simulink model "water_hopper_fix"  (Simulink 7.9)
settings: Solver=ode23t  StartTime=0.0  StopTime=5  MaxStep=1e-3  RelTol=1e-3
values from neighbouring files (symbols this model uses):
  Amp = AMP(jj,1)    [TwoD_search.m]
  C_d = 0.703    [SimParam.m]
  density = 1000    [SimParam.m]
  freq = FREQ(1,kk)    [TwoD_search.m]
  g = 9.81    [SimParam.m]
  h0 = leg_length    [TwoD_search.m]
  leg_length = 0.06    [SimParam.m]
  mass = 0.05    [SimParam.m]
  S1 = pi*r1^2    (= 0.00125663706144)    [SimParam.m]
  S2 = pi*r2^2    (= 7.85398163397e-05)    [SimParam.m]
libraries: mblibv1 x13, simulink x1
settings Model: Creator=Metti  LastModifiedBy=Metti
settings SolverCC: ZeroCrossControl=DisableAll
settings ConfigurationSet: Description=SimMechanics 2G

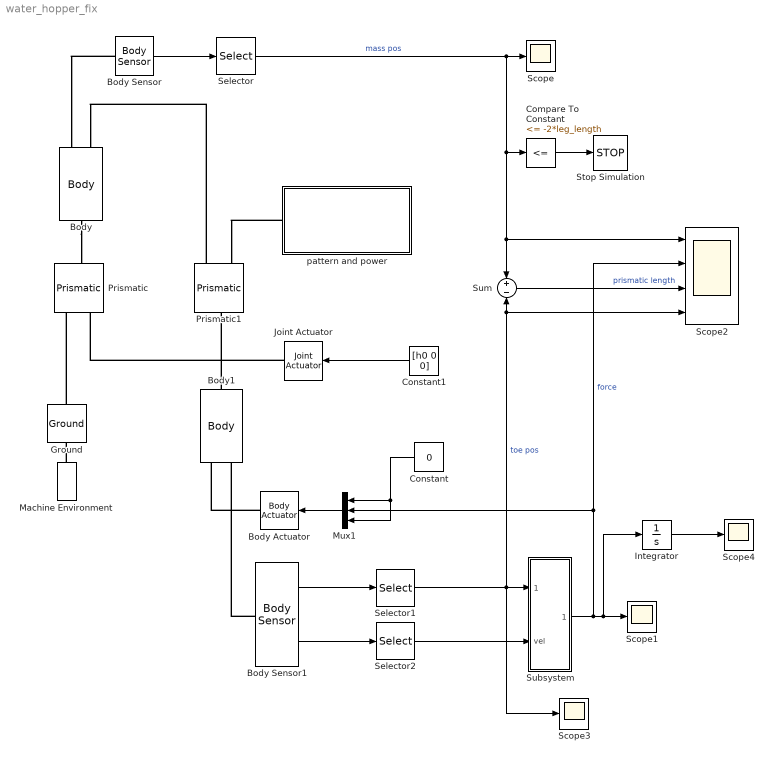
== system water_hopper_fix ==
  Body : mblibv1/Bodies/Body  LConnTagsString=CS1  RConnTagsString=CS2|CS3  UpdateFromCAD=off  DialogClass=MechanicalBodyBlock  Mass=mass  MassUnits=kg  InertiaUnits=kg*m^2  Inertia=eye(3)  Shape=Cylinder  ShapeDims=[1 1]  ShapeUnits=m  ShapeUse=false  Density=1  DensityUnits=kg/m^3  DensityUse=false  GraphicsMode=MACHINE_DEFAULT  BodyColorSelMode=MACHINE_DEFAULT  BodyColor=[1 0 0]  AttachedToCS=CG  CG=Left$CG$[0 0 0]$WORLD$WORLD$m$[0 0 0]$Euler X-Y-Z$deg$WORLD$false$none  WorkingFrames=Left$CS1$[0 0 0]$CG$CG$m$[0 0 0]$Euler X-Y-Z$deg$WORLD$true$none#Right$CS2$[0 0 0]$CG$CG$m$[0 0 0]$Euler X-Y-Z$deg$WORLD$true$none#Right$CS3$[0 0 0]$CG$CG$m$[0 0 0]$Euler X-Y-Z$deg$WORLD$true$none  CGPos=[0 0 0]  CGRot=[0 0 0]  CS0Pos=[]  CS0Rot=[]  CS1Pos=[0 0 0]  CS1Rot=[0 0 0]  CS2Pos=[0 0 0]  CS2Rot=[0 0 0]  CS3Pos=[0 0 0]  CS3Rot=[0 0 0]  CS4Pos=[]  CS4Rot=[]  CS5Pos=[]  CS5Rot=[]  CS6Pos=[]  CS6Rot=[]  CS7Pos=[]  CS7Rot=[]  CS8Pos=[]  CS8Rot=[]  CS9Pos=[]  CS9Rot=[]  CS10Pos=[]  CS10Rot=[]  CS11Pos=[]  CS11Rot=[]  CS12Pos=[]  CS12Rot=[]  CS13Pos=[]  CS13Rot=[]  CS14Pos=[]  CS14Rot=[]  CS15Pos=[]  CS15Rot=[]  CS16Pos=[]  CS16Rot=[]  CS17Pos=[]  CS17Rot=[]  CS18Pos=[]  CS18Rot=[]  CS19Pos=[]  CS19Rot=[]  CS20Pos=[]  CS20Rot=[]
  Body Actuator : mblibv1/Sensors &  Actuators/Body Actuator  UpdateFromCAD=off  PhysicalDomain=Mechanical  PortType=blob  ActuationStyle=Force  AngleUnits=deg  ArcVelocityUnits=deg/s  ArcAccelerationUnits=deg/s^2  CoordPositionUnits=m  VelocityUnits=m/s  AccelerationUnits=m/s^2  ForceUnits=N  TorqueUnits=N-m  ActiveIO=on  Width=3  DialogClass=MechanicalActuatorBlock  ReferenceFrame=Absolute (World)  Angle=off  CoordPosition=on  Force=on  Torque=off
  Body Sensor : mblibv1/Sensors &  Actuators/Body Sensor  UpdateFromCAD=off  PhysicalDomain=Mechanical  PortType=blob  Muxed=on  Pose=off  Angle=on  AngleUnits=deg  ArcVelocity=off  ArcVelocityUnits=deg/s  ArcAcceleration=off  ArcAccelerationUnits=deg/s^2  CoordPosition=on  CoordPositionUnits=m  Velocity=off  VelocityUnits=m/s  Acceleration=off  AccelerationUnits=m/s^2  Quaternion=on  QuaternionDT=off  QuaternionDDT=off  QuaternionUnits=off  OutputVector=[1]  ActiveIO=on  Width=3  DialogClass=MechanicalSensorBlock  ReferenceFrame=Absolute (World)
  Body Sensor1 : mblibv1/Sensors &  Actuators/Body Sensor  UpdateFromCAD=off  PhysicalDomain=Mechanical  PortType=blob  Muxed=off  Pose=off  Angle=on  AngleUnits=deg  ArcVelocity=off  ArcVelocityUnits=deg/s  ArcAcceleration=off  ArcAccelerationUnits=deg/s^2  CoordPosition=on  CoordPositionUnits=m  Velocity=on  VelocityUnits=m/s  Acceleration=off  AccelerationUnits=m/s^2  Quaternion=on  QuaternionDT=off  QuaternionDDT=off  QuaternionUnits=off  OutputVector=[1]  ActiveIO=on  Width=6  DialogClass=MechanicalSensorBlock  ReferenceFrame=Absolute (World)
  Body1 : mblibv1/Bodies/Body  LConnTagsString=CS1  RConnTagsString=CS2|CS3  UpdateFromCAD=off  DialogClass=MechanicalBodyBlock  Mass=0  MassUnits=kg  InertiaUnits=kg*m^2  Inertia=eye(3)  Shape=Cylinder  ShapeDims=[1 1]  ShapeUnits=m  ShapeUse=false  Density=1  DensityUnits=kg/m^3  DensityUse=false  GraphicsMode=MACHINE_DEFAULT  BodyColorSelMode=MACHINE_DEFAULT  BodyColor=[1 0 0]  AttachedToCS=CG  CG=Left$CG$[0 -leg_length 0]$CS1$CS1$m$[0 0 0]$Euler X-Y-Z$deg$WORLD$false$none  WorkingFrames=Left$CS1$[0 0 0]$Adjoining$Adjoining$m$[0 0 0]$Euler X-Y-Z$deg$WORLD$true$none#Right$CS2$[0 -leg_length 0]$CS1$CS1$m$[0 0 0]$Euler X-Y-Z$deg$WORLD$true$none#Right$CS3$[0 -leg_length 0]$CS1$CS1$m$[0 0 0]$Euler X-Y-Z$deg$WORLD$true$none  CGPos=[0 -leg_length 0]  CGRot=[0 0 0]  CS0Pos=[]  CS0Rot=[]  CS1Pos=[0 0 0]  CS1Rot=[0 0 0]  CS2Pos=[0 -leg_length 0]  CS2Rot=[0 0 0]  CS3Pos=[0 -leg_length 0]  CS3Rot=[0 0 0]  CS4Pos=[]  CS4Rot=[]  CS5Pos=[]  CS5Rot=[]  CS6Pos=[]  CS6Rot=[]  CS7Pos=[]  CS7Rot=[]  CS8Pos=[]  CS8Rot=[]  CS9Pos=[]  CS9Rot=[]  CS10Pos=[]  CS10Rot=[]  CS11Pos=[]  CS11Rot=[]  CS12Pos=[]  CS12Rot=[]  CS13Pos=[]  CS13Rot=[]  CS14Pos=[]  CS14Rot=[]  CS15Pos=[]  CS15Rot=[]  CS16Pos=[]  CS16Rot=[]  CS17Pos=[]  CS17Rot=[]  CS18Pos=[]  CS18Rot=[]  CS19Pos=[]  CS19Rot=[]  CS20Pos=[]  CS20Rot=[]
  Compare To Constant : simulink/Logic and Bit Operations/Compare To Constant  relop=<=  const=-2*leg_length  OutDataTypeStr=boolean
  Constant : Constant  Value=0
  Constant1 : Constant  Value=[h0 0 0]
  Ground : mblibv1/Bodies/Ground  UpdateFromCAD=off  LeftPortType=env  RightPortType=workingframe  PhysicalDomain=Mechanical  DialogClass=GroundBlock  CoordPosition=[0 0 0]  CoordPositionUnits=m  StateVectorMgrId=3  MachineId=[3 0]  ShowEnvPort=on
  Integrator : Integrator
  Joint Actuator : mblibv1/Sensors &  Actuators/Joint Actuator  UpdateFromCAD=off  PhysicalDomain=Mechanical  PortType=blob  ActuationStyle=Motion  AngleUnits=deg  ArcVelocityUnits=deg/s  ArcAccelerationUnits=deg/s^2  CoordPositionUnits=m  VelocityUnits=m/s  AccelerationUnits=m/s^2  ForceUnits=N  TorqueUnits=N*m  ActiveIO=on  Width=3  DialogClass=MechanicalActuatorBlock  Primitive=P1  ReferenceFrame=Absolute (World)
  Machine Environment : mblibv1/Bodies/Machine Environment  PortType=env  PhysicalDomain=Mechanical  DialogTemplateClass=MECH.MachineEnvironment  SyncWhenCopied=off  Gravity=[0 -g 0]  GravityUnits=m/s^2  GravityAsSignal=off  Dimensionality=Auto-detect  AnalysisType=Forward dynamics  LinearAssemblyTolerance=1e-3  LinearAssemblyToleranceUnits=m  AngularAssemblyTolerance=1e-3  AngularAssemblyToleranceUnits=rad  ConstraintSolverType=Stabilizing  ConstraintRelTolerance=1e-4  ConstraintAbsTolerance=1e-4  UseRobustSingularityHandling=off  RedundancyAnalysisToleranceType=Automatically select tolerance  RedundancyAnalysisTolerance=1e-14  StatePerturbationType=Fixed  PerturbationSize=1e-5  VisualizeMachine=on  BodyVisualizationType=Use model default body geometries  BodyColorSelMode=Use model default  DefaultBodyColor=[1 0 0]
  Mux1 : Mux  Inputs=3
  Prismatic : mblibv1/Joints/Prismatic  LConnTagsString=__newl0|SA1  RConnTagsString=__newr0  UpdateFromCAD=off  NumSAPorts=1  CutJoint=off  MarkAsCut=off  Primitives=prismatic  PrimitiveProps=P1$World$[0 1 0]$prismatic  DialogClass=JointBlock  P1Axis=[0 1 0]
  Prismatic1 : mblibv1/Joints/Prismatic  LConnTagsString=__newl0|SA1  RConnTagsString=__newr0  UpdateFromCAD=off  NumSAPorts=1  CutJoint=off  MarkAsCut=off  Primitives=prismatic  PrimitiveProps=P1$World$[0 1 0]$prismatic  DialogClass=JointBlock  P1Axis=[0 1 0]
  Scope{,1,3..4} (4 alike) : Scope
      Scope settings: YMin=-0.053045  YMax=-0.053005  SaveName=ball_position
      Scope1 settings: SaveName=force
      Scope3 settings: SaveName=toe_position
      Scope4 settings: SaveName=Int_Force
  Scope2 : Scope  NumInputPorts=4
      settings: YMin=-5~-5~-5~-5  YMax=5~5~5~5  SaveName=ScopeData2
  Selector : Selector  InputPortWidth=3  IndexOptions=Index vector (dialog)  Indices=[2]  OutputSizes=1
  Selector1 : Selector  InputPortWidth=3  IndexOptions=Index vector (dialog)  Indices=[2]  OutputSizes=1
  Selector2 : Selector  InputPortWidth=3  IndexOptions=Index vector (dialog)  Indices=[2]  OutputSizes=1
  Stop Simulation : Stop
  Subsystem : Subsystem
  Sum : Sum  Inputs=+|-
  pattern and power : Subsystem
  wires:
  Body Sensor/1 -> Selector/1
  Selector/1 -> Scope/1, Scope2/1, Sum/1, Compare To Constant/1  "mass pos"
  Body Sensor1/1 -> Selector1/1
  Body Sensor1/2 -> Selector2/1
  Selector1/1 -> Sum/2, Scope2/4, Subsystem/1(pos), Scope3/1  "toe pos"
  Selector2/1 -> Subsystem/2(vel)
  Subsystem/1(force) -> Mux1/2, Scope2/2, Scope1/1, Integrator/1  "force"
  Mux1/1 -> Body Actuator/1
  Constant/1 -> Mux1/1, Mux1/3
  Sum/1 -> Scope2/3  "prismatic length"
  Compare To Constant/1 -> Stop Simulation/1
  Constant1/1 -> Joint Actuator/1
  Integrator/1 -> Scope4/1
  connections:
  Body Sensor/LConn1 -- Body/RConn1
  Body/LConn1 -- Prismatic/RConn1
  Machine Environment/RConn1 -- Ground/LConn1
  Ground/RConn1 -- Prismatic/LConn1
  Body1/LConn1 -- Prismatic1/RConn1
  Body Actuator/RConn1 -- Body1/RConn1
  Body Sensor1/LConn1 -- Body1/RConn2
  Prismatic1/LConn1 -- Body/RConn2
  Joint Actuator/RConn1 -- Prismatic/LConn2
  pattern and power/LConn1 -- Prismatic1/LConn2

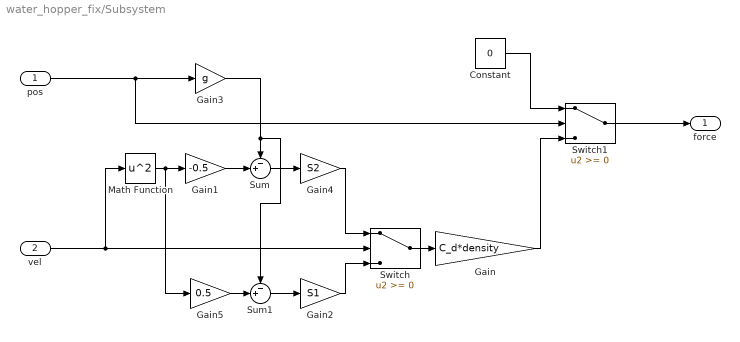
== system water_hopper_fix/Subsystem ==
  pos : Inport
  vel : Inport  Port=2
  Constant : Constant  Value=0
  Gain : Gain  Gain=C_d*density
  Gain1 : Gain  Gain=-0.5
  Gain2 : Gain  Gain=S1
  Gain3 : Gain  Gain=g
  Gain4 : Gain  Gain=S2
  Gain5 : Gain  Gain=0.5
  Math Function : Math  Operator=square  SaturateOnIntegerOverflow=on
  Sum : Sum  Inputs=-+|
  Sum1 : Sum  Inputs=-+|
  Switch : Switch  ZeroCross=off
  Switch1 : Switch
  force : Outport
  wires:
  vel/1 -> Switch/2, Math Function/1
  Math Function/1 -> Gain1/1, Gain5/1
  Gain1/1 -> Sum/2
  pos/1 -> Gain3/1, Switch1/2
  Gain3/1 -> Sum/1, Sum1/1
  Sum/1 -> Gain4/1
  Gain4/1 -> Switch/1
  Gain2/1 -> Switch/3
  Switch/1 -> Gain/1
  Switch1/1 -> force/1
  Gain/1 -> Switch1/3
  Constant/1 -> Switch1/1
  Sum1/1 -> Gain2/1
  Gain5/1 -> Sum1/2

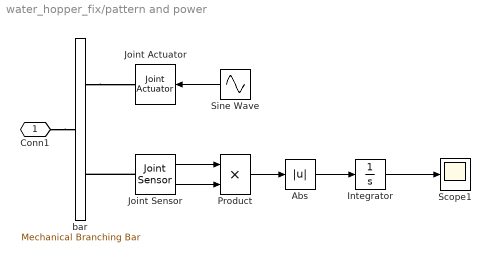
== system water_hopper_fix/pattern and power ==
  Abs : Abs
  Integrator : Integrator
  Joint Actuator : mblibv1/Sensors &  Actuators/Joint Actuator  UpdateFromCAD=off  PhysicalDomain=Mechanical  PortType=blob  ActuationStyle=Motion  AngleUnits=deg  ArcVelocityUnits=deg/s  ArcAccelerationUnits=deg/s^2  CoordPositionUnits=m  VelocityUnits=m/s  AccelerationUnits=m/s^2  ForceUnits=N  TorqueUnits=N*m  ActiveIO=on  Width=3  DialogClass=MechanicalActuatorBlock  Primitive=P1  ReferenceFrame=Absolute (World)
  Joint Sensor : mblibv1/Sensors &  Actuators/Joint Sensor  UpdateFromCAD=off  PhysicalDomain=Mechanical  PortType=blob  Muxed=off  Pose=off  Angle=on  AngleUnits=deg  ArcVelocity=off  ArcVelocityUnits=deg/s  ArcAcceleration=off  ArcAccelerationUnits=deg/s^2  CoordPosition=off  CoordPositionUnits=m  Velocity=on  VelocityUnits=m/s  Acceleration=off  AccelerationUnits=m/s^2  Quaternion=on  QuaternionDT=off  QuaternionDDT=off  QuaternionUnits=off  OutputVector=[1]  ActiveIO=on  Width=2  DialogClass=MechanicalSensorBlock  Primitive=P1  Force=on  ForceUnits=N  Torque=off  TorqueUnits=N*m  ReferenceFrame=Absolute (World)  ReactionSensedSide=Base  ReactionReferenceFrame=Absolute (World)  ReactionForce=off  ReactionForceUnits=N  ReactionMoment=off  ReactionMomentUnits=N*m
  Product : Product  RndMeth=Zero
  Scope1 : Scope
      settings: SaveName=Work
  Sine Wave : Sin  Amplitude=[Amp Amp*freq -Amp*freq^2]  Frequency=freq  Phase=[0 pi/2 0]  SampleTime=0
  bar : mblibv1/Utilities/Mechanical Branching Bar  LConnTagsString=_newl0  RConnTagsString=SA0|SA1  UpdateFromCAD=off  DialogClass=MechanicalBranchingBarBlock  NumSAPorts=2
  Conn1 : PMIOPort  Port=1  Side=Left
  wires:
  Sine Wave/1 -> Joint Actuator/1
  Joint Sensor/1 -> Product/1
  Product/1 -> Abs/1
  Abs/1 -> Integrator/1
  Integrator/1 -> Scope1/1
  Joint Sensor/2 -> Product/2
  connections:
  bar/RConn1 -- Joint Actuator/RConn1
  Joint Sensor/LConn1 -- bar/RConn2
  Conn1/RConn1 -- bar/LConn1
